simulink model "L2"  (R2024a)
settings: Solver=FixedStepAuto  StartTime=0.0  StopTime=time_end  FixedStep=time_sampling  MaxStep=0.01  RelTol=1e-3
values from neighbouring files (symbols this model uses):
  err_max = 0.3 * pi/2    (= 0.471238898038)    [main.m]
  freq_L3_max = 15    [main.m]
  freq_L3_min = -15    [main.m]
  gain_coup = 1.6    [main.m]
  incidence_mat = full(incidence(my_graph))    [main.m]
  index_L2 = 4    [main.m]
  omega_n = [3.04, 6.36, 3.34, 9.91, 5.21]'    [main.m]
  speed_thres_ascending = 1    [main.m]
  speed_thres_descending = 2.5    [main.m]
  theta_0 = zeros(n_particip, 1)    [main.m]
  thres_max = 1 * pi/2    (= 1.57079632679)    [main.m]
  thres_min = 0.3 * pi/2    (= 0.471238898038)    [main.m]
  time_sampling = 0.01    [main.m]
libraries: dspstat3 x3, deeplib x1
settings Model: PacingRate=0.089000  Creator=marco  LastModifiedBy=marco
settings RTWCC: GPUComputeCapability=3.5

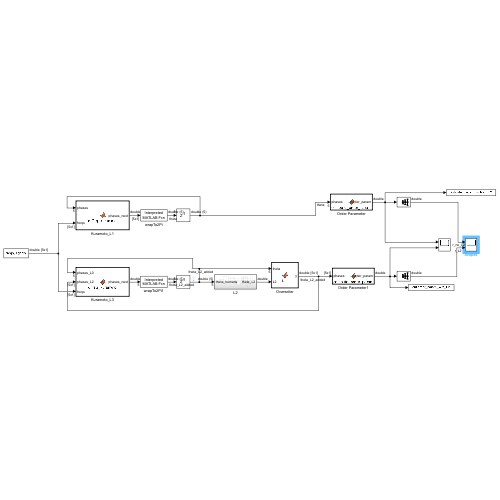
[thumbnail: Simulink's stored preview of the top-level diagram]
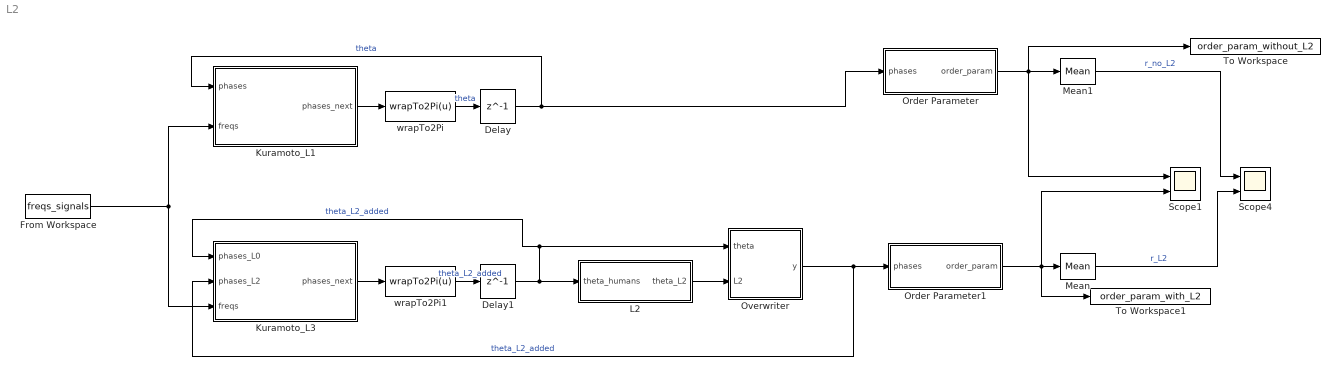
== system L2 ==
  Delay : Delay  DelayLength=1  InitialCondition=theta_0
  Delay1 : Delay  DelayLength=1  InitialCondition=theta_0
  From Workspace : FromWorkspace  VariableName=freqs_signals  Interpolate=off  OutputAfterFinalValue=Holding final value
  Kuramoto_L1 : MATLAB Function  TreatAsAtomicUnit=on
  Kuramoto_L3 : MATLAB Function  TreatAsAtomicUnit=on
  L2 : Subsystem
  Mean : dspstat3/Mean  run=on  InputProcessing=Columns as channels (frame based)  reset_popup=None  directionMode=Each column  dimension=1  roiEnable=off  roiType=Rectangles  roiPortion=Entire ROI  roiOutput=Individual statistics for each ROI  roiFlag=off  roundingMode=Floor  overflowMode=off  outputDataTypeStr=Inherit: Same as accumulator  outputMin=[]  outputMax=[]  outputLastDataTypeStr=Inherit: Same as accumulator
  Mean1 : dspstat3/Mean  run=on  InputProcessing=Columns as channels (frame based)  reset_popup=None  directionMode=Each column  dimension=1  roiEnable=off  roiType=Rectangles  roiPortion=Entire ROI  roiOutput=Individual statistics for each ROI  roiFlag=off  roundingMode=Floor  overflowMode=off  outputDataTypeStr=Inherit: Same as accumulator  outputMin=[]  outputMax=[]  outputLastDataTypeStr=Inherit: Same as accumulator
  Order Parameter : MATLAB Function  TreatAsAtomicUnit=on
  Order Parameter1 : MATLAB Function  TreatAsAtomicUnit=on
  Overwriter : MATLAB Function  TreatAsAtomicUnit=on
  Scope1 : Scope  NumInputPorts=2
  Scope4 : Scope  NumInputPorts=2
  To Workspace : ToWorkspace  VariableName=order_param_without_L2  SaveFormat=Timeseries  SampleTime=-1
  To Workspace1 : ToWorkspace  VariableName=order_param_with_L2  SaveFormat=Timeseries  SampleTime=-1
  wrapTo2Pi : MATLABFcn  MATLABFcn=wrapTo2Pi(u)
  wrapTo2Pi1 : MATLABFcn  MATLABFcn=wrapTo2Pi(u)
  wires:
  Mean1/1 -> Scope4/1  "r_no_L2"
  Mean/1 -> Scope4/2  "r_L2"
  From Workspace/1 -> Kuramoto_L1/2(freqs), Kuramoto_L3/3(freqs)
  Delay1/1 -> Overwriter/1(theta), Kuramoto_L3/1(phases_L0), L2/1(theta_humans)  "theta_L2_added"
  Order Parameter1/1(order_param) -> To Workspace1/1, Scope1/2, Mean/1
  Delay/1 -> Order Parameter/1(phases), Kuramoto_L1/1(phases)  "theta"
  L2/1(theta_L2) -> Overwriter/2(L2)
  Order Parameter/1(order_param) -> To Workspace/1, Scope1/1, Mean1/1
  Kuramoto_L1/1(phases_next) -> wrapTo2Pi/1
  Kuramoto_L3/1(phases_next) -> wrapTo2Pi1/1
  wrapTo2Pi/1 -> Delay/1  "theta"
  wrapTo2Pi1/1 -> Delay1/1  "theta_L2_added"
  Overwriter/1(y) -> Kuramoto_L3/2(phases_L2), Order Parameter1/1(phases)  "theta_L2_added"

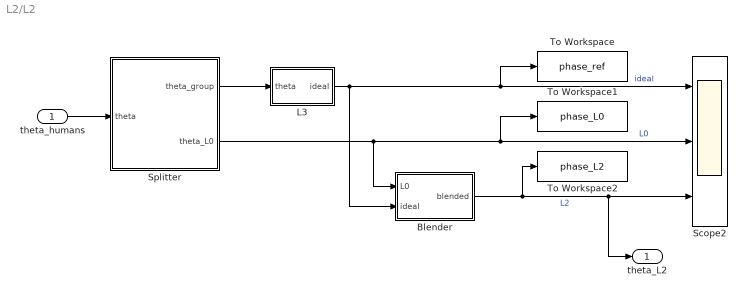
== system L2/L2 ==
  theta_humans : Inport
  Blender : Subsystem
  L3 : Subsystem
  Scope2 : Scope  NumInputPorts=3
  Splitter : MATLAB Function  TreatAsAtomicUnit=on
  To Workspace : ToWorkspace  VariableName=phase_ref  SaveFormat=Timeseries  SampleTime=-1
  To Workspace1 : ToWorkspace  VariableName=phase_L0  SaveFormat=Timeseries  SampleTime=-1
  To Workspace2 : ToWorkspace  VariableName=phase_L2  SaveFormat=Timeseries  SampleTime=-1
  theta_L2 : Outport
  wires:
  Splitter/2(theta_L0) -> Blender/1(L0), To Workspace1/1, Scope2/2  "L0"
  Blender/1(blended) -> theta_L2/1, Scope2/3, To Workspace2/1  "L2"
  L3/1(ideal) -> Blender/2(ideal), To Workspace/1, Scope2/1  "ideal"
  theta_humans/1 -> Splitter/1(theta)
  Splitter/1(theta_group) -> L3/1(theta)

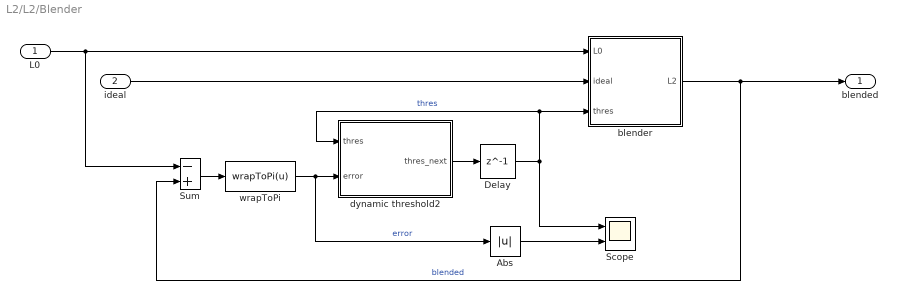
== system L2/L2/Blender ==
  L0 : Inport
  ideal : Inport  Port=2
  Abs : Abs  SaturateOnIntegerOverflow=off
  Delay : Delay  DelayLength=1  InitialCondition=thres_max
  Scope : Scope  NumInputPorts=2
  Sum : Sum  Inputs=-+
  blender : MATLAB Function  TreatAsAtomicUnit=on
  dynamic threshold2 : MATLAB Function  TreatAsAtomicUnit=on
  wrapToPi : MATLABFcn  MATLABFcn=wrapToPi(u)
  blended : Outport
  wires:
  blender/1(L2) -> Sum/2, blended/1  "blended"
  ideal/1 -> blender/2(ideal)
  wrapToPi/1 -> Abs/1, dynamic threshold2/2(error)  "error"
  L0/1 -> Sum/1, blender/1(L0)
  Delay/1 -> blender/3(thres), dynamic threshold2/1(thres), Scope/1  "thres"
  dynamic threshold2/1(thres_next) -> Delay/1
  Abs/1 -> Scope/2
  Sum/1 -> wrapToPi/1

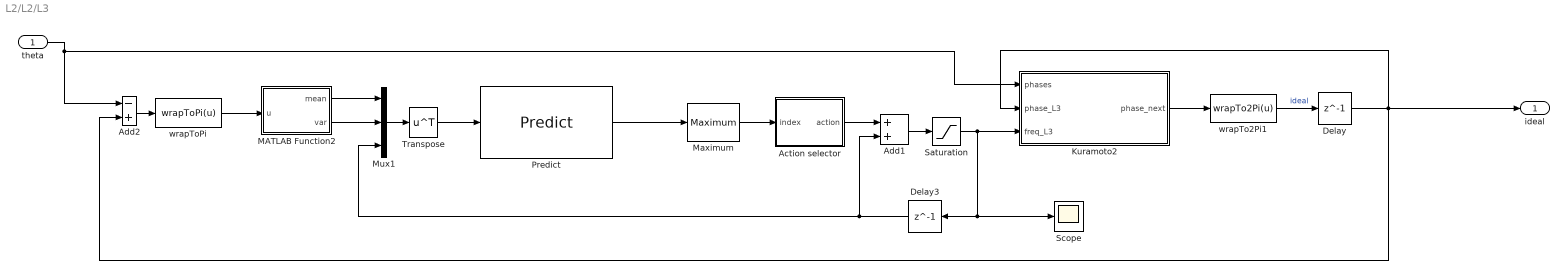
== system L2/L2/L3 ==
  theta : Inport
  Action selector : MATLAB Function  TreatAsAtomicUnit=on
  Add1 : Sum
  Add2 : Sum  Inputs=-+
  Delay : Delay  DelayLength=1  InitialCondition=theta_0(index_L2)
  Delay3 : Delay  DelayLength=1  InitialCondition=mean(omega_n)
  Kuramoto2 : MATLAB Function  TreatAsAtomicUnit=on
  MATLAB Function2 : MATLAB Function  TreatAsAtomicUnit=on
  Maximum : dspstat3/Maximum  operation=maximum  fcn=Index  indexBase=One  operateOver=Each column  Dimension=1  InputProcessing=Columns as channels (frame based)  reset=None  roiEnable=off  roiType=Rectangles  roiPortion=Entire ROI  roiOutput=Individual statistics for each ROI  roiFlag=off  roundingMode=Floor  overflowMode=off  accumDataTypeStr=Inherit: Same as product output  accumLastDataTypeStr=Inherit: Same as product output
      settings: LibrarySourceBlock=dsphdlsupportstat/Maximum
  Mux1 : Mux  Inputs=3
  Predict : deeplib/Predict  Network=Network from MAT-file  NetworkFunction=squeezenet  NetworkFilePath=L3.mat  MiniBatchSize=128  InputDataFormats={ 'input_1', 'BC' }  Predictions=on  Activations={}  ForceInterpretedSim=off  EnableDLNetwork=on  LastKnownNetworkFilePath='L3.mat'  LastKnownNetworkTimeStamp=739410.529814814799465239048004150390625
  Saturation : Saturate  UpperLimit=freq_L3_max  LowerLimit=freq_L3_min
  Scope : Scope
  Transpose : Math  Operator=transpose
  wrapTo2Pi1 : MATLABFcn  MATLABFcn=wrapTo2Pi(u)
  wrapToPi : MATLABFcn  MATLABFcn=wrapToPi(u)
  ideal : Outport
  wires:
  Predict/1 -> Maximum/1
  Add1/1 -> Saturation/1
  MATLAB Function2/1(mean) -> Mux1/1
  Maximum/1 -> Action selector/1(index)
  Delay3/1 -> Mux1/3, Add1/2
  MATLAB Function2/2(var) -> Mux1/2
  wrapToPi/1 -> MATLAB Function2/1(u)
  Transpose/1 -> Predict/1
  Saturation/1 -> Kuramoto2/3(freq_L3), Scope/1, Delay3/1
  Mux1/1 -> Transpose/1
  Action selector/1(action) -> Add1/1
  theta/1 -> Kuramoto2/1(phases), Add2/1
  Add2/1 -> wrapToPi/1
  Delay/1 -> Add2/2, Kuramoto2/2(phase_L3), ideal/1
  Kuramoto2/1(phase_next) -> wrapTo2Pi1/1
  wrapTo2Pi1/1 -> Delay/1  "ideal"

== matlab function L2/Blender/dynamic threshold2 ==
  data: thres input; error input; thres_max parameter; thres_min parameter; thres_next output; speed_thres_ascending parameter; speed_thres_descending parameter; time_sampling parameter; err_max parameter
function thres_next = thres_dyn(thres, error, thres_max, thres_min, speed_thres_ascending, speed_thres_descending, time_sampling, err_max)    

    % steady_state_val = test_fun(error/err_max) * (thres_max-thres_min) + thres_min;
    steady_state_val = triang_fun(error/err_max) * (thres_max-thres_min) + thres_min;
    if thres <= steady_state_val
        thres_next = thres + time_sampling * (- speed_thres_ascending * (thres - steady_state_val));
    else
        thres_next = thres + time_sampling * (- speed_thres_descending * (thres - steady_state_val));
    end
end

== matlab function L2/Blender/blender ==
  data: L0 input; L2 output; ideal input; thres input; p_norm parameter
function L2 = blender(L0, ideal, thres, p_norm)
   
% saturated_input = sat_smooth(wrapToPi(ideal - L0), thres, p_norm);
saturated_input = sat_hard(wrapToPi(ideal - L0), thres);
L2              = wrapTo2Pi(L0 + saturated_input);
end

function y = sat_smooth(x, thres, p)
    y = x / ((1 + abs(x /thres)^p)^(1/p));
end

function y = sat_hard(x, thres)
    if x >= thres 
        y = thres;
    elseif x <= - thres 
        y = - thres;
    else
        y = x;
    end
end

== matlab function L2/Order Parameter ==
  data: phases input; order_param output
function order_param = compute_order_param(phases)

order_param = compute_order_param(phases);

end

== matlab function L2/Order Parameter1 ==
  data: phases input; order_param output
function order_param = compute_order_param(phases)

order_param = compute_order_param(phases);

end

== matlab function L2/Splitter ==
  data: theta input; theta_group output; theta_L0 output; index_L2 parameter
function [theta_group, theta_L0] = fcn(theta, index_L2)

% n = length(theta);
% indices_group = [1:index_L2-1, index_L2+1:n]';
% theta_group = theta(indices_group);
% theta_L0 = theta(index_L2);

n = length(theta);
theta_group = theta(1:n-1);
theta_L0 = 0;
count = 1;
for i = 1:n
    if i ~= index_L2
        theta_group(count) = theta(i);
        count=count+1;
    else
        theta_L0 = theta(i);
    end
end

== matlab function L2/Overwriter ==
  data: theta input; y output; L2 input; index_L2 parameter
function y = fcn(theta, L2,index_L2)
y = theta;
y(index_L2) = L2;

== matlab function L2/L3/Action selector ==
  data: index input; action output; action_space_L3 parameter
function action = fcn(index, action_space_L3)

action = action_space_L3(index);

end

== matlab function L2/Kuramoto_L1 ==
  data: phases input; freqs input; gain_coup parameter; phases_next output; incidence_mat parameter; time_sampling parameter
function phases_next = diffeq_kuramoto(phases, freqs, gain_coup, incidence_mat, time_sampling)

phases_next = diffeq_kuramoto(phases, freqs, gain_coup, incidence_mat, time_sampling);

end

== matlab function L2/L3/MATLAB Function2 ==
  data: u input; mean output; var output
function [mean, var] = fcn(u)

q = sum(exp(1i * u))/length(u);
mean = angle(q);
var = 1-abs(q);

== matlab function L2/L3/Kuramoto2 ==
  data: phases input; phase_L3 input; phase_next output; gain_coup parameter; freq_L3 input; time_sampling parameter; incidence_mat parameter; index_L2 parameter; omega_n parameter
function phase_next = kuramoto_fn(phases, phase_L3, gain_coup, freq_L3, time_sampling, incidence_mat, index_L2, omega_n)

phases = [phases(1:index_L2-1); phase_L3; phases(index_L2:end)];
phase_next = phase_L3 + time_sampling * (freq_L3 + gain_coup * incidence_mat(index_L2, :) * sin (- incidence_mat' * phases));

end

== matlab function L2/Kuramoto_L3 ==
  data: phases_L0 input; phases_L2 input; freqs input; gain_coup parameter; phases_next output; incidence_mat parameter; time_sampling parameter
function phases_next = diffeq_kuramoto(phases_L0, phases_L2, freqs, gain_coup, incidence_mat, time_sampling)

phases_next = phases_L0 + time_sampling * (freqs + gain_coup * incidence_mat * sin (- incidence_mat' * phases_L2));


end
